simulink model "hex_simplify_mono"  (R2017a)
settings: Solver=VariableStepAuto  StartTime=0.0  StopTime=30  RelTol=1e-3
model workspace: external: MATLAB File C:\Users\laure\Documents\Gonzalo\Robotica-II\hexapod-robot\simscape\simplify_model\hex_DataFile1.m (data not in the file)
undefined symbols (not defined in the file): sigbuilder_block, smiData, X, Y, Z
libraries: sm_lib x20, nesl_utility x19
settings Model: Creator=laure  LastModifiedBy=laure

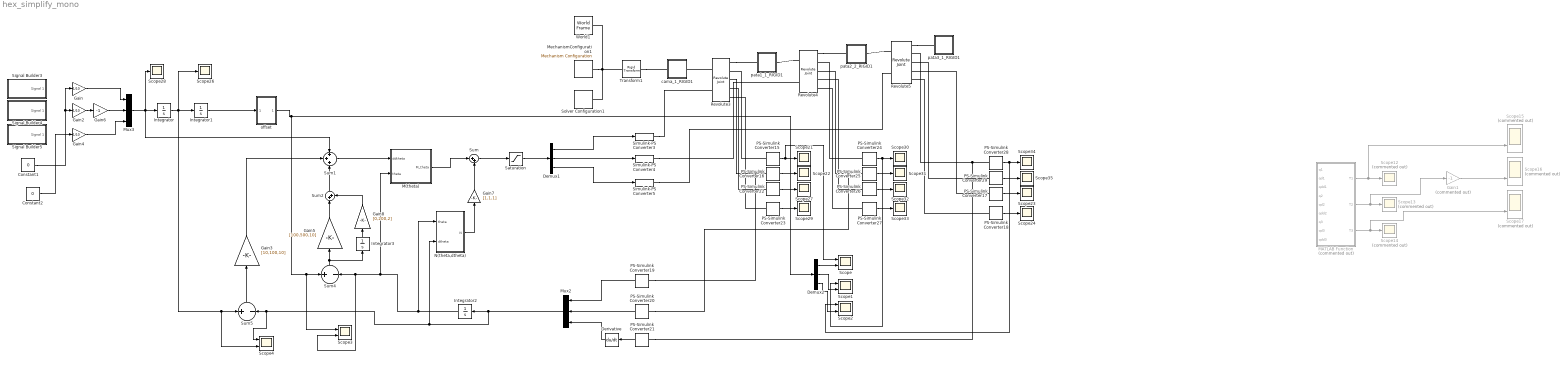
== system hex_simplify_mono ==
  Constant1 : Constant  Value=0
  Constant2 : Constant  Value=0
  Demux1 : Demux  Outputs=3
  Demux2 : Demux  Outputs=3
  Derivative : Derivative
  Gain : Gain  Gain=1/10
  Gain1 : Gain  Commented=on  Gain=-1
  Gain2 : Gain  Gain=1/10
  Gain3 : Gain  Gain=[10,100,10]
  Gain4 : Gain  Gain=1/10
  Gain5 : Gain  Gain=[100,500,10]
  Gain6 : Gain  Gain=-1
  Gain7 : Gain  Gain=[1,1,1]
  Gain8 : Gain  Gain=[0,200,2]
  Integrator : Integrator
  Integrator1 : Integrator
  Integrator2 : Integrator  InitialCondition=[-pi/2 - pi/6,-pi/2,pi/2]
  Integrator3 : Integrator  InitialCondition=[-pi/2 - pi/6,-pi/2,pi/2]
  M(theta) : Subsystem
  MATLAB Function : MATLAB Function  Commented=on  TreatAsAtomicUnit=on
  MechanismConfiguration1 : sm_lib/Utilities/Mechanism Configuration  UniformGravity=Constant  GravityVector=[0 0 -9.81]  GravityUnits=m/s^2  LinearizationDelta=0.001
  Mux2 : Mux  Inputs=3
  Mux3 : Mux  Inputs=3
  N(theta,dtheta) : Subsystem
  PS-Simulink Converter{15..29} (15 alike) : nesl_utility/PS-Simulink Converter  PhysicalDomain=network_engine_domain  SubClassName=ps_output  LeftPortType=input  RightPortType=output  PseudoPeriodic=off  Frequencies=[]  Unit=1  AffineConversion=off
  Revolute3 : sm_lib/Joints/Revolute Joint  SenseConstraintForce=off  SenseConstraintForceX=off  SenseConstraintForceY=off  SenseConstraintForceZ=off  SenseConstraintTorque=off  SenseConstraintTorqueX=off  SenseConstraintTorqueY=off  SenseConstraintTorqueZ=off  SenseTotalForce=off  SenseTotalForceX=off  SenseTotalForceY=off  SenseTotalForceZ=off  SenseTotalTorque=off  SenseTotalTorqueX=off  SenseTotalTorqueY=off  SenseTotalTorqueZ=off  CompositeWrenchDir=FollowerOnBase  CompositeWrenchFrame=BaseFrame  EquilibriumPosition=0  EquilibriumPositionUnits=rad  SpringStiffness=0  SpringStiffnessUnits=N*m/rad  DampingCoefficient=0.1  DampingCoefficientUnits=N*m/(rad/s)  TorqueActuationMode=InputTorque  MotionActuationMode=ComputedMotion  SensePosition=on  SenseVelocity=on  SenseAcceleration=on  SenseTorqueForce=on  PositionTargetSpecify=on  PositionTargetPriority=Low  PositionTargetValue=-pi/2 - pi/6  PositionTargetValueUnits=rad  VelocityTargetSpecify=off  VelocityTargetPriority=High  VelocityTargetValue=0  VelocityTargetValueUnits=deg/s
  Revolute4 : sm_lib/Joints/Revolute Joint  SenseConstraintForce=off  SenseConstraintForceX=off  SenseConstraintForceY=off  SenseConstraintForceZ=off  SenseConstraintTorque=off  SenseConstraintTorqueX=off  SenseConstraintTorqueY=off  SenseConstraintTorqueZ=off  SenseTotalForce=off  SenseTotalForceX=off  SenseTotalForceY=off  SenseTotalForceZ=off  SenseTotalTorque=off  SenseTotalTorqueX=off  SenseTotalTorqueY=off  SenseTotalTorqueZ=off  CompositeWrenchDir=FollowerOnBase  CompositeWrenchFrame=BaseFrame  EquilibriumPosition=0  EquilibriumPositionUnits=rad  SpringStiffness=0  SpringStiffnessUnits=N*m/rad  DampingCoefficient=0.1  DampingCoefficientUnits=N*m/(rad/s)  TorqueActuationMode=InputTorque  MotionActuationMode=ComputedMotion  SensePosition=on  SenseVelocity=on  SenseAcceleration=on  SenseTorqueForce=on  PositionTargetSpecify=on  PositionTargetPriority=Low  PositionTargetValue=-pi/2  PositionTargetValueUnits=rad  VelocityTargetSpecify=on  VelocityTargetPriority=High  VelocityTargetValue=0  VelocityTargetValueUnits=deg/s
  Revolute5 : sm_lib/Joints/Revolute Joint  SenseConstraintForce=off  SenseConstraintForceX=off  SenseConstraintForceY=off  SenseConstraintForceZ=off  SenseConstraintTorque=off  SenseConstraintTorqueX=off  SenseConstraintTorqueY=off  SenseConstraintTorqueZ=off  SenseTotalForce=off  SenseTotalForceX=off  SenseTotalForceY=off  SenseTotalForceZ=off  SenseTotalTorque=off  SenseTotalTorqueX=off  SenseTotalTorqueY=off  SenseTotalTorqueZ=off  CompositeWrenchDir=FollowerOnBase  CompositeWrenchFrame=BaseFrame  EquilibriumPosition=0  EquilibriumPositionUnits=rad  SpringStiffness=0  SpringStiffnessUnits=N*m/rad  DampingCoefficient=0.1  DampingCoefficientUnits=N*m/(rad/s)  TorqueActuationMode=InputTorque  MotionActuationMode=ComputedMotion  SensePosition=on  SenseVelocity=on  SenseAcceleration=on  SenseTorqueForce=on  PositionTargetSpecify=on  PositionTargetPriority=Low  PositionTargetValue=pi/2  PositionTargetValueUnits=rad  VelocityTargetSpecify=off  VelocityTargetPriority=High  VelocityTargetValue=0  VelocityTargetValueUnits=deg/s
  Saturation : Saturate  UpperLimit=5  LowerLimit=-5  LinearizeAsGain=off  ZeroCross=off
  Scope{,1..4} (5 alike) : Scope  NumInputPorts=2
  Scope12 : Scope  Commented=on
  Scope13 : Scope  Commented=on
  Scope14 : Scope  Commented=on
  Scope15 : Scope  Commented=on  NumInputPorts=2
  Scope16 : Scope  Commented=on  NumInputPorts=2
  Scope17 : Scope  Commented=on  NumInputPorts=2
  Scope{21..24,26..35} (14 alike) : Scope
  Signal Builder3 : Subsystem  Tag=STV Subsys  LoadFcn=sigbuilder_block('load');  StartFcn=sigbuilder_block('start');  StopFcn=sigbuilder_block('stop');  ClipboardFcn=sigbuilder_block('clipboard');  mask(Sigbuilder block){tuvar=[0:10]}
      mask help: Simulink:masks:SigbuilderBlock_MD
      mask init:
      | if ~strcmp(get_param(bdroot(gcbh),'SimulationStatus'),'stopped') tuvar = sigbuilder_block('maskInit'); end
      settings: CopyFcn=sigbuilder_block('copy');  DeleteFcn=sigbuilder_block('delete');  ModelCloseFcn=sigbuilder_block('modelClose');  PreSaveFcn=sigbuilder_block('preSave');  PauseFcn=sigbuilder_block('pause');  ContinueFcn=sigbuilder_block('continue');  NameChangeFcn=sigbuilder_block('namechange');  OpenFcn=sigbuilder_block('open',[319.5 111 550.5 359.25 ]);  CloseFcn=sigbuilder_block('close');
      mask Display: plot(0, 0, 100, 100,[2, 2, 32, 32, 2], [68, 8, 8, 68, 68],[32, 2], [38, 38], [32, 19, 2],[53, 60, 44], [32, 17, 17, 2],[16, 16, 31, 31]);txt = getActiveGroup(gcbh);text(2, 100, txt,'verticalAlignment', 'top');
  Signal Builder4 : Subsystem  Tag=STV Subsys  LoadFcn=sigbuilder_block('load');  StartFcn=sigbuilder_block('start');  StopFcn=sigbuilder_block('stop');  ClipboardFcn=sigbuilder_block('clipboard');  mask(Sigbuilder block){tuvar=[0:10]}
      mask help: Simulink:masks:SigbuilderBlock_MD
      mask init:
      | if ~strcmp(get_param(bdroot(gcbh),'SimulationStatus'),'stopped') tuvar = sigbuilder_block('maskInit'); end
      settings: CopyFcn=sigbuilder_block('copy');  DeleteFcn=sigbuilder_block('delete');  ModelCloseFcn=sigbuilder_block('modelClose');  PreSaveFcn=sigbuilder_block('preSave');  PauseFcn=sigbuilder_block('pause');  ContinueFcn=sigbuilder_block('continue');  NameChangeFcn=sigbuilder_block('namechange');  OpenFcn=sigbuilder_block('open',[319.5 111 550.5 359.25 ]);  CloseFcn=sigbuilder_block('close');
      mask Display: plot(0, 0, 100, 100,[2, 2, 32, 32, 2], [68, 8, 8, 68, 68],[32, 2], [38, 38], [32, 19, 2],[53, 60, 44], [32, 17, 17, 2],[16, 16, 31, 31]);txt = getActiveGroup(gcbh);text(2, 100, txt,'verticalAlignment', 'top');
  Signal Builder5 : Subsystem  Tag=STV Subsys  LoadFcn=sigbuilder_block('load');  StartFcn=sigbuilder_block('start');  StopFcn=sigbuilder_block('stop');  ClipboardFcn=sigbuilder_block('clipboard');  mask(Sigbuilder block){tuvar=[0:10]}
      mask help: Simulink:masks:SigbuilderBlock_MD
      mask init:
      | if ~strcmp(get_param(bdroot(gcbh),'SimulationStatus'),'stopped') tuvar = sigbuilder_block('maskInit'); end
      settings: CopyFcn=sigbuilder_block('copy');  DeleteFcn=sigbuilder_block('delete');  ModelCloseFcn=sigbuilder_block('modelClose');  PreSaveFcn=sigbuilder_block('preSave');  PauseFcn=sigbuilder_block('pause');  ContinueFcn=sigbuilder_block('continue');  NameChangeFcn=sigbuilder_block('namechange');  OpenFcn=sigbuilder_block('open',[319.5 111 550.5 359.25 ]);  CloseFcn=sigbuilder_block('close');
      mask Display: plot(0, 0, 100, 100,[2, 2, 32, 32, 2], [68, 8, 8, 68, 68],[32, 2], [38, 38], [32, 19, 2],[53, 60, 44], [32, 17, 17, 2],[16, 16, 31, 31]);txt = getActiveGroup(gcbh);text(2, 100, txt,'verticalAlignment', 'top');
  Simulink-PS Converter3 : nesl_utility/Simulink-PS Converter  PhysicalDomain=network_engine_domain  SubClassName=ps_input  LeftPortType=input  RightPortType=output  PseudoPeriodic=off  Frequencies=[]  NoiseDistribution=none  NoiseParameters=[]  Unit=1  AffineConversion=off  FilteringAndDerivatives=filter  SimscapeFilterOrder=2  InputFilterTimeConstant=0.001  UdotUserProvided=0
  Simulink-PS Converter4 : nesl_utility/Simulink-PS Converter  PhysicalDomain=network_engine_domain  SubClassName=ps_input  LeftPortType=input  RightPortType=output  PseudoPeriodic=off  Frequencies=[]  NoiseDistribution=none  NoiseParameters=[]  Unit=1  AffineConversion=off  FilteringAndDerivatives=filter  SimscapeFilterOrder=2  InputFilterTimeConstant=0.001  UdotUserProvided=0
  Simulink-PS Converter5 : nesl_utility/Simulink-PS Converter  PhysicalDomain=network_engine_domain  SubClassName=ps_input  LeftPortType=input  RightPortType=output  PseudoPeriodic=off  Frequencies=[]  NoiseDistribution=none  NoiseParameters=[]  Unit=1  AffineConversion=off  FilteringAndDerivatives=filter  SimscapeFilterOrder=2  InputFilterTimeConstant=0.001  UdotUserProvided=0
  Solver Configuration1 : nesl_utility/Solver Configuration  PhysicalDomain=network_engine_domain  SubClassName=solver  LeftPortType=input  RightPortType=generic  Accelerate=off  Tones=[]  Harmonics=[]  SimulateNoise=off  Profile=off  UseLocalSampling=off  EnableSwitchedLinearOptims=on  FrequencyDomain=off  UseCCode=off  RelTol=0.001  AbsTol=1e-06  MinStep=1e-09  ToWorkspace=off  RevertToSquareIcSolve=off  NumHomotopyIterations=100  PhasorMode=off  PhasorModeNumHarmonics=1  OverrideAbsTol=off  DoDC=off  ResidualTolerance=1e-09  UseLocalSolver=off  LocalSolverChoice=NE_BACKWARD_EULER_ADVANCER  LocalSolverSampleTime=0.001  DoFixedCost=off  MaxNonlinIter=3  MaxModeIter=2  LinearAlgebra=Sparse  DelaysMemoryBudget=1024  AutomaticFiltering=on  FilteringTimeConstant=0.001
  Sum : Sum  Inputs=|++
  Sum1 : Sum  Inputs=+++
  Sum2 : Sum  Inputs=|++
  Sum4 : Sum  Inputs=+-
  Sum5 : Sum  Inputs=+-
  Transform1 : sm_lib/Frames and Transforms/Rigid Transform  TranslationMethod=Cartesian  TranslationStandardOffset=0  TranslationLengthUnit=mm  TranslationStandardAxis=+Z  TranslationCartesianOffset=smiData.RigidTransform(7).translation  TranslationROffset=0  TranslationROffsetUnits=m  TranslationZOffset=0  TranslationZOffsetUnits=m  TranslationThetaOffset=0  TranslationThetaOffsetUnits=deg  RotationMethod=ArbitraryAxis  RotationAngleUnits=rad  RotationStandardAxis=+Z  RotationAngle=smiData.RigidTransform(7).angle  RotationArbitraryAxis=smiData.RigidTransform(7).axis  FollAlignAxisA=+X  BaseAlignAxisA=+Y  FollAlignAxisB=+Y  BaseAlignAxisB=+Z  RotationSequenceAxes=FollowerAxes  RotationSequence=XYX  RotationSequenceAngles=[0 0 0]  RotationSequenceAnglesUnits=deg  RotationMatrix=[1 0 0; 0 1 0; 0 0 1]
  World1 : sm_lib/Frames and Transforms/World Frame
  cama_1_RIGID1 : Subsystem
  "offset " : Subsystem
  pata1_1_RIGID1 : Subsystem
  pata2_2_RIGID1 : Subsystem
  pata3_1_RIGID1 : Subsystem
  wires:
  MATLAB Function/1(T1) -> Scope15/2, Scope12/1
  MATLAB Function/3(T3) -> Scope17/2, Scope14/1
  MATLAB Function/2(T2) -> Gain1/1, Scope13/1
  Gain1/1 -> Scope16/2
  Gain6/1 -> Mux3/2
  Sum5/1 -> Gain3/1
  Gain/1 -> Mux3/1
  Integrator1/1 -> "offset "/1(In1)
  PS-Simulink Converter19/1 -> Mux2/1
  PS-Simulink Converter21/1 -> Derivative/1
  Mux3/1 -> Sum1/1, Integrator/1, Scope28/1
  PS-Simulink Converter18/1 -> Scope24/1
  PS-Simulink Converter28/1 -> Scope2/1, Scope34/1
  Sum4/1 -> Gain5/1, Integrator3/1
  PS-Simulink Converter29/1 -> Scope35/1
  PS-Simulink Converter25/1 -> Scope31/1
  PS-Simulink Converter20/1 -> Mux2/2
  PS-Simulink Converter24/1 -> Scope1/1, Scope30/1
  PS-Simulink Converter26/1 -> Scope32/1
  Integrator/1 -> Integrator1/1, Scope4/2, Sum5/1, Scope26/1
  PS-Simulink Converter27/1 -> Scope33/1
  PS-Simulink Converter16/1 -> Scope22/1
  PS-Simulink Converter23/1 -> Scope29/1
  PS-Simulink Converter22/1 -> Scope27/1
  Gain4/1 -> Mux3/3
  PS-Simulink Converter15/1 -> Scope/1, Scope21/1
  PS-Simulink Converter17/1 -> Scope23/1
  Gain2/1 -> Gain6/1
  "offset "/1(Out1) -> Scope3/1, Sum4/1, Demux2/1
  Sum/1 -> Saturation/1
  N(theta,dtheta)/1(N) -> Gain7/1
  Gain3/1 -> Sum1/2
  Demux2/1 -> Scope/2
  Demux2/2 -> Scope1/2
  Demux2/3 -> Scope2/2
  Sum1/1 -> M(theta)/1(ddtheta)
  M(theta)/1(M_theta) -> Sum/1
  Gain7/1 -> Sum/2
  Mux2/1 -> N(theta,dtheta)/2(dtheta), Scope4/1, Sum5/2, Integrator2/1
  Integrator2/1 -> N(theta,dtheta)/1(theta), M(theta)/2(theta), Scope3/2, Sum4/2
  Demux1/1 -> Simulink-PS Converter3/1
  Demux1/2 -> Simulink-PS Converter4/1
  Sum2/1 -> Sum1/3
  Gain5/1 -> Sum2/1
  Integrator3/1 -> Gain8/1
  Gain8/1 -> Sum2/2
  Derivative/1 -> Mux2/3
  Saturation/1 -> Demux1/1
  Demux1/3 -> Simulink-PS Converter5/1
  Constant1/1 -> Gain2/1, Gain/1
  Constant2/1 -> Gain4/1
  connections:
  World1/RConn1 -- Transform1/LConn1 -- MechanismConfiguration1/RConn1 -- Solver Configuration1/RConn1
  PS-Simulink Converter28/LConn1 -- PS-Simulink Converter21/LConn1 -- Revolute5/RConn2
  PS-Simulink Converter15/LConn1 -- Revolute3/RConn2
  PS-Simulink Converter24/LConn1 -- Revolute4/RConn2
  Revolute4/RConn1 -- pata2_2_RIGID1/LConn1
  PS-Simulink Converter22/LConn1 -- Revolute3/RConn4
  PS-Simulink Converter17/LConn1 -- Revolute5/RConn4
  Transform1/RConn1 -- cama_1_RIGID1/LConn1
  PS-Simulink Converter23/LConn1 -- Revolute3/RConn5
  Simulink-PS Converter5/RConn1 -- Revolute5/LConn2
  PS-Simulink Converter25/LConn1 -- PS-Simulink Converter20/LConn1 -- Revolute4/RConn3
  PS-Simulink Converter27/LConn1 -- Revolute4/RConn5
  PS-Simulink Converter26/LConn1 -- Revolute4/RConn4
  Revolute3/LConn1 -- cama_1_RIGID1/RConn1
  Revolute4/LConn1 -- pata1_1_RIGID1/RConn1
  Revolute5/RConn1 -- pata3_1_RIGID1/LConn1
  Revolute5/LConn1 -- pata2_2_RIGID1/RConn1
  Simulink-PS Converter3/RConn1 -- Revolute3/LConn2
  PS-Simulink Converter18/LConn1 -- Revolute5/RConn5
  PS-Simulink Converter29/LConn1 -- Revolute5/RConn3
  Simulink-PS Converter4/RConn1 -- Revolute4/LConn2
  Revolute3/RConn1 -- pata1_1_RIGID1/LConn1
  Revolute3/RConn3 -- PS-Simulink Converter19/LConn1 -- PS-Simulink Converter16/LConn1

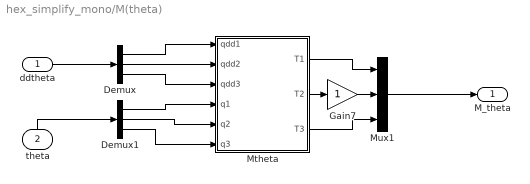
== system hex_simplify_mono/M(theta) ==
  ddtheta : Inport
  theta : Inport  Port=2
  Demux : Demux  Outputs=3
  Demux1 : Demux  Outputs=3
  Gain7 : Gain
  Mtheta : MATLAB Function  TreatAsAtomicUnit=on
  Mux1 : Mux  Inputs=3
  M_theta : Outport
  wires:
  Mux1/1 -> M_theta/1
  Mtheta/3(T3) -> Mux1/3
  Mtheta/2(T2) -> Gain7/1
  Mtheta/1(T1) -> Mux1/1
  Gain7/1 -> Mux1/2
  ddtheta/1 -> Demux/1
  theta/1 -> Demux1/1
  Demux/2 -> Mtheta/2(qdd2)
  Demux/1 -> Mtheta/1(qdd1)
  Demux/3 -> Mtheta/3(qdd3)
  Demux1/1 -> Mtheta/4(q1)
  Demux1/2 -> Mtheta/5(q2)
  Demux1/3 -> Mtheta/6(q3)

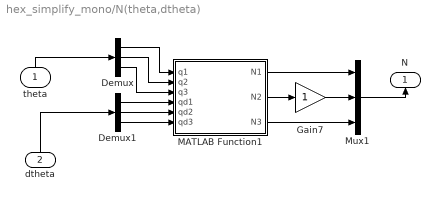
== system hex_simplify_mono/N(theta,dtheta) ==
  theta : Inport
  dtheta : Inport  Port=2
  Demux : Demux  Outputs=3
  Demux1 : Demux  Outputs=3
  Gain7 : Gain
  MATLAB Function1 : MATLAB Function  TreatAsAtomicUnit=on
  Mux1 : Mux  Inputs=3
  N : Outport
  wires:
  MATLAB Function1/3(N3) -> Mux1/3
  MATLAB Function1/1(N1) -> Mux1/1
  Mux1/1 -> N/1
  MATLAB Function1/2(N2) -> Gain7/1
  theta/1 -> Demux/1
  dtheta/1 -> Demux1/1
  Demux/1 -> MATLAB Function1/1(q1)
  Demux/2 -> MATLAB Function1/2(q2)
  Demux/3 -> MATLAB Function1/3(q3)
  Demux1/1 -> MATLAB Function1/4(qd1)
  Demux1/2 -> MATLAB Function1/5(qd2)
  Demux1/3 -> MATLAB Function1/6(qd3)
  Gain7/1 -> Mux1/2

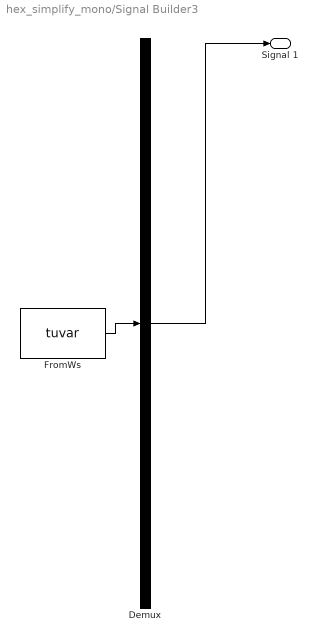
== system hex_simplify_mono/Signal Builder3 ==
  Demux : Demux  Tag=STV Demux  Outputs=1
  FromWs : FromWorkspace  Tag=STV FromWs  VariableName=tuvar  SampleTime=0
      SigBuilderData=|
      | common.afterFinalStr = 'Extrapolate'
      | common.sampleTime = 0
      | dataSet.timeRange = [0 10]
      | dataSet.name = 'Group 1'
      | sbobj.Groups.Name = 'Group 1'
      | sbobj.Groups.Signals.Name = 'Signal 1'
      | sbobj.Groups.Signals.XData = [0 4 6 10]
      | sbobj.Groups.Signals.YData = [0 1.57079632679 1.57079632679 0]
  Signal 1 : Outport  Tag=STV Outport
  wires:
  Demux/1 -> Signal 1/1
  FromWs/1 -> Demux/1

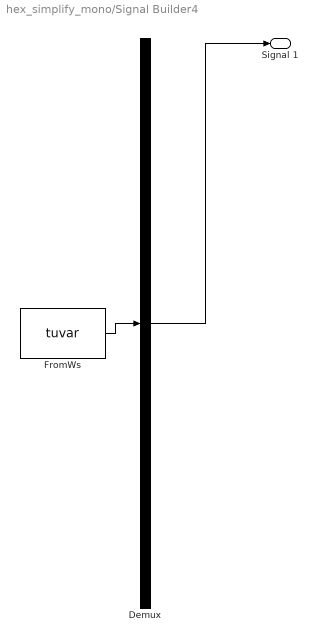
== system hex_simplify_mono/Signal Builder4 ==
  Demux : Demux  Tag=STV Demux  Outputs=1
  FromWs : FromWorkspace  Tag=STV FromWs  VariableName=tuvar  SampleTime=0
      SigBuilderData=|
      | common.afterFinalStr = 'Extrapolate'
      | common.sampleTime = 0
      | dataSet.timeRange = [0 10]
      | dataSet.name = 'Group 1'
      | sbobj.Groups.Name = 'Group 1'
      | sbobj.Groups.Signals.Name = 'Signal 1'
      | sbobj.Groups.Signals.XData = [0 4 6 10]
      | sbobj.Groups.Signals.YData = [0 1.57079632679 1.57079632679 0]
  Signal 1 : Outport  Tag=STV Outport
  wires:
  Demux/1 -> Signal 1/1
  FromWs/1 -> Demux/1

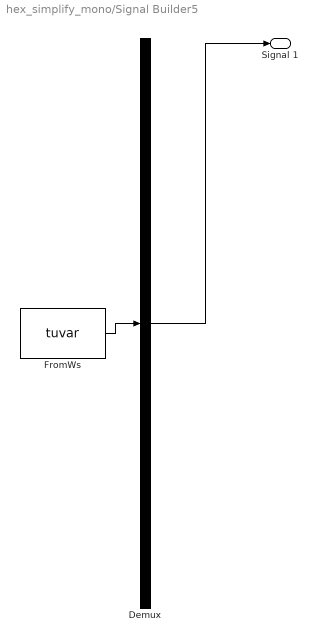
== system hex_simplify_mono/Signal Builder5 ==
  Demux : Demux  Tag=STV Demux  Outputs=1
  FromWs : FromWorkspace  Tag=STV FromWs  VariableName=tuvar  SampleTime=0
      SigBuilderData=|
      | common.afterFinalStr = 'Extrapolate'
      | common.sampleTime = 0
      | dataSet.timeRange = [0 10]
      | dataSet.name = 'Group 1'
      | sbobj.Groups.Name = 'Group 1'
      | sbobj.Groups.Signals.Name = 'Signal 1'
      | sbobj.Groups.Signals.XData = [0 4 6 10]
      | sbobj.Groups.Signals.YData = [0 1.57079632679 1.57079632679 0]
  Signal 1 : Outport  Tag=STV Outport
  wires:
  Demux/1 -> Signal 1/1
  FromWs/1 -> Demux/1

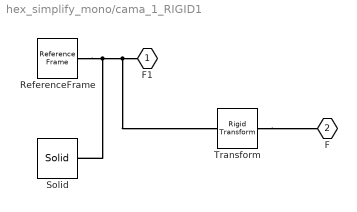
== system hex_simplify_mono/cama_1_RIGID1 ==
  ReferenceFrame : sm_lib/Frames and Transforms/Reference Frame
  Solid : sm_lib/Body Elements/Solid  InertiaType=Custom  Mass=smiData.Solid(2).mass  MassUnits=kg  CenterOfMass=smiData.Solid(2).CoM  CenterOfMassUnits=mm  MomentsOfInertia=smiData.Solid(2).MoI  MomentsOfInertiaUnits=kg*mm^2  ProductsOfInertia=smiData.Solid(2).PoI  ProductsOfInertiaUnits=kg*mm^2  DensityBased=on  Density=1000  DensityUnits=kg/m^3  DoExposeReferenceFrame=on  SerializedFrames=<Frames/>  GraphicType=FromGeometry  MarkerShape=Sphere  MarkerSize=10  GraphicVisPropType=SimpleVisualProperties  GraphicDiffuseColor=smiData.Solid(2).color  GraphicSpecularColor=[0.5 0.5 0.5 1.0]  GraphicAmbientColor=[0.15 0.15 0.15 1.0]  GraphicEmissiveColor=[0.0 0.0 0.0 1.0]  GraphicShininess=75  GraphicOpacity=smiData.Solid(2).opacity  GeometryShape=FromFile  RectangleSize=[1 1]  RectangleSizeUnits=m  BrickDimensions=[1 1 1]  BrickDimensionUnits=m  CylinderRadius=1  CylinderRadiusUnits=m  CylinderLength=1  CylinderLengthUnits=m  SphereRadius=1  SphereRadiusUnits=m  EllipsoidRadii=[1 1 1]  EllipsoidRadiiUnits=m  ExtrusionCrossSection=[1 1; -1 1; -1 -1; 1 -1]  ExtrusionCrossSectionUnits=m  ExtrusionLength=1  ExtrusionLengthUnits=m  PolygonNumSides=3  PolygonOuterRadius=1  PolygonOuterRadiusUnits=m  ExtGeomFileType=STEP  ExtGeomFileName=cama_Predeterminado_sldprt.STEP  ExtGeomFileUnits=m  RevolutionCrossSection=[1 1; 1 -1; 2 -1; 2 1]  RevolutionCrossSectionUnits=m  RevolutionExtent=Full  RevolutionAngle=180  RevolutionAngleUnits=deg
  Transform : sm_lib/Frames and Transforms/Rigid Transform  TranslationMethod=Cartesian  TranslationStandardOffset=0  TranslationLengthUnit=mm  TranslationStandardAxis=+Z  TranslationCartesianOffset=smiData.RigidTransform(1).translation  TranslationROffset=0  TranslationROffsetUnits=m  TranslationZOffset=0  TranslationZOffsetUnits=m  TranslationThetaOffset=0  TranslationThetaOffsetUnits=deg  RotationMethod=ArbitraryAxis  RotationAngleUnits=rad  RotationStandardAxis=+Z  RotationAngle=smiData.RigidTransform(1).angle  RotationArbitraryAxis=smiData.RigidTransform(1).axis  FollAlignAxisA=+X  BaseAlignAxisA=+Y  FollAlignAxisB=+Y  BaseAlignAxisB=+Z  RotationSequenceAxes=FollowerAxes  RotationSequence=XYX  RotationSequenceAngles=[0 0 0]  RotationSequenceAnglesUnits=deg  RotationMatrix=[1 0 0; 0 1 0; 0 0 1]
  F1 : PMIOPort  Port=1  Side=Left
  F : PMIOPort  Port=2  Side=Right
  connections:
  Solid/RConn1 -- ReferenceFrame/RConn1 -- Transform/LConn1 -- F1/RConn1
  Transform/RConn1 -- F/RConn1

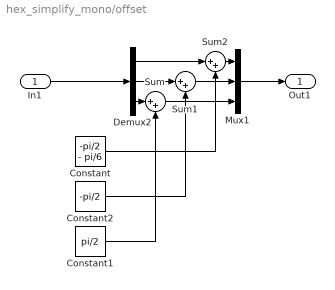
== system hex_simplify_mono/offset  ==
  In1 : Inport
  Constant : Constant  Value=-pi/2 - pi/6
  Constant1 : Constant  Value=pi/2
  Constant2 : Constant  Value=-pi/2
  Demux2 : Demux  Outputs=3
  Mux1 : Mux  Inputs=3
  Sum : Sum  Inputs=|++
  Sum1 : Sum  Inputs=|++
  Sum2 : Sum  Inputs=|++
  Out1 : Outport
  wires:
  Mux1/1 -> Out1/1
  In1/1 -> Demux2/1
  Sum/1 -> Mux1/3
  Demux2/3 -> Sum/1
  Sum1/1 -> Mux1/2
  Demux2/2 -> Sum1/1
  Sum2/1 -> Mux1/1
  Demux2/1 -> Sum2/1
  Constant/1 -> Sum2/2
  Constant2/1 -> Sum1/2
  Constant1/1 -> Sum/2

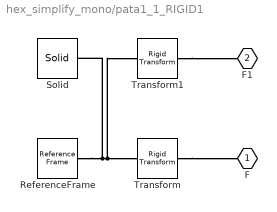
== system hex_simplify_mono/pata1_1_RIGID1 ==
  ReferenceFrame : sm_lib/Frames and Transforms/Reference Frame
  Solid : sm_lib/Body Elements/Solid  InertiaType=Custom  Mass=2  MassUnits=kg  CenterOfMass=[24.25,7.5,-7.5]  CenterOfMassUnits=mm  MomentsOfInertia=[0,0,0]  MomentsOfInertiaUnits=kg*mm^2  ProductsOfInertia=[0,0,0]  ProductsOfInertiaUnits=kg*mm^2  DensityBased=on  Density=1000  DensityUnits=kg/m^3  DoExposeReferenceFrame=on  SerializedFrames=<Frames/>  GraphicType=FromGeometry  MarkerShape=Sphere  MarkerSize=10  GraphicVisPropType=SimpleVisualProperties  GraphicDiffuseColor=smiData.Solid(4).color  GraphicSpecularColor=[0.5 0.5 0.5 1.0]  GraphicAmbientColor=[0.15 0.15 0.15 1.0]  GraphicEmissiveColor=[0.0 0.0 0.0 1.0]  GraphicShininess=75  GraphicOpacity=smiData.Solid(4).opacity  GeometryShape=FromFile  RectangleSize=[1 1]  RectangleSizeUnits=m  BrickDimensions=[1 1 1]  BrickDimensionUnits=m  CylinderRadius=1  CylinderRadiusUnits=m  CylinderLength=1  CylinderLengthUnits=m  SphereRadius=1  SphereRadiusUnits=m  EllipsoidRadii=[1 1 1]  EllipsoidRadiiUnits=m  ExtrusionCrossSection=[1 1; -1 1; -1 -1; 1 -1]  ExtrusionCrossSectionUnits=m  ExtrusionLength=1  ExtrusionLengthUnits=m  PolygonNumSides=3  PolygonOuterRadius=1  PolygonOuterRadiusUnits=m  ExtGeomFileType=STEP  ExtGeomFileName=pata1_Predeterminado_sldprt.STEP  ExtGeomFileUnits=m  RevolutionCrossSection=[1 1; 1 -1; 2 -1; 2 1]  RevolutionCrossSectionUnits=m  RevolutionExtent=Full  RevolutionAngle=180  RevolutionAngleUnits=deg
  Transform : sm_lib/Frames and Transforms/Rigid Transform  TranslationMethod=Cartesian  TranslationStandardOffset=0  TranslationLengthUnit=mm  TranslationStandardAxis=+Z  TranslationCartesianOffset=smiData.RigidTransform(2).translation  TranslationROffset=0  TranslationROffsetUnits=m  TranslationZOffset=0  TranslationZOffsetUnits=m  TranslationThetaOffset=0  TranslationThetaOffsetUnits=deg  RotationMethod=ArbitraryAxis  RotationAngleUnits=rad  RotationStandardAxis=+Z  RotationAngle=smiData.RigidTransform(2).angle  RotationArbitraryAxis=smiData.RigidTransform(2).axis  FollAlignAxisA=+X  BaseAlignAxisA=+Y  FollAlignAxisB=+Y  BaseAlignAxisB=+Z  RotationSequenceAxes=FollowerAxes  RotationSequence=XYX  RotationSequenceAngles=[0 0 0]  RotationSequenceAnglesUnits=deg  RotationMatrix=[1 0 0; 0 1 0; 0 0 1]
  Transform1 : sm_lib/Frames and Transforms/Rigid Transform  TranslationMethod=Cartesian  TranslationStandardOffset=0  TranslationLengthUnit=mm  TranslationStandardAxis=+Z  TranslationCartesianOffset=smiData.RigidTransform(3).translation  TranslationROffset=0  TranslationROffsetUnits=m  TranslationZOffset=0  TranslationZOffsetUnits=m  TranslationThetaOffset=0  TranslationThetaOffsetUnits=deg  RotationMethod=ArbitraryAxis  RotationAngleUnits=rad  RotationStandardAxis=+Z  RotationAngle=smiData.RigidTransform(3).angle  RotationArbitraryAxis=smiData.RigidTransform(3).axis  FollAlignAxisA=+X  BaseAlignAxisA=+Y  FollAlignAxisB=+Y  BaseAlignAxisB=+Z  RotationSequenceAxes=FollowerAxes  RotationSequence=XYX  RotationSequenceAngles=[0 0 0]  RotationSequenceAnglesUnits=deg  RotationMatrix=[1 0 0; 0 1 0; 0 0 1]
  F : PMIOPort  Port=1  Side=Left
  F1 : PMIOPort  Port=2  Side=Right
  connections:
  Solid/RConn1 -- ReferenceFrame/RConn1 -- Transform/LConn1 -- Transform1/LConn1
  Transform/RConn1 -- F/RConn1
  Transform1/RConn1 -- F1/RConn1

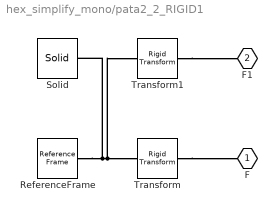
== system hex_simplify_mono/pata2_2_RIGID1 ==
  ReferenceFrame : sm_lib/Frames and Transforms/Reference Frame
  Solid : sm_lib/Body Elements/Solid  InertiaType=Custom  Mass=2  MassUnits=kg  CenterOfMass=[47.9, 7.5, 12.5]  CenterOfMassUnits=mm  MomentsOfInertia=[0,0,0]  MomentsOfInertiaUnits=kg*mm^2  ProductsOfInertia=[0,0,0]  ProductsOfInertiaUnits=kg*mm^2  DensityBased=on  Density=1000  DensityUnits=kg/m^3  DoExposeReferenceFrame=on  SerializedFrames=<Frames/>  GraphicType=FromGeometry  MarkerShape=Sphere  MarkerSize=10  GraphicVisPropType=SimpleVisualProperties  GraphicDiffuseColor=smiData.Solid(3).color  GraphicSpecularColor=[0.5 0.5 0.5 1.0]  GraphicAmbientColor=[0.15 0.15 0.15 1.0]  GraphicEmissiveColor=[0.0 0.0 0.0 1.0]  GraphicShininess=75  GraphicOpacity=smiData.Solid(3).opacity  GeometryShape=FromFile  RectangleSize=[1 1]  RectangleSizeUnits=m  BrickDimensions=[1 1 1]  BrickDimensionUnits=m  CylinderRadius=1  CylinderRadiusUnits=m  CylinderLength=1  CylinderLengthUnits=m  SphereRadius=1  SphereRadiusUnits=m  EllipsoidRadii=[1 1 1]  EllipsoidRadiiUnits=m  ExtrusionCrossSection=[1 1; -1 1; -1 -1; 1 -1]  ExtrusionCrossSectionUnits=m  ExtrusionLength=1  ExtrusionLengthUnits=m  PolygonNumSides=3  PolygonOuterRadius=1  PolygonOuterRadiusUnits=m  ExtGeomFileType=STEP  ExtGeomFileName=pata2_Predeterminado_sldprt.STEP  ExtGeomFileUnits=m  RevolutionCrossSection=[1 1; 1 -1; 2 -1; 2 1]  RevolutionCrossSectionUnits=m  RevolutionExtent=Full  RevolutionAngle=180  RevolutionAngleUnits=deg
  Transform : sm_lib/Frames and Transforms/Rigid Transform  TranslationMethod=Cartesian  TranslationStandardOffset=0  TranslationLengthUnit=mm  TranslationStandardAxis=+Z  TranslationCartesianOffset=smiData.RigidTransform(4).translation  TranslationROffset=0  TranslationROffsetUnits=m  TranslationZOffset=0  TranslationZOffsetUnits=m  TranslationThetaOffset=0  TranslationThetaOffsetUnits=deg  RotationMethod=ArbitraryAxis  RotationAngleUnits=rad  RotationStandardAxis=+Z  RotationAngle=smiData.RigidTransform(4).angle  RotationArbitraryAxis=smiData.RigidTransform(4).axis  FollAlignAxisA=+X  BaseAlignAxisA=+Y  FollAlignAxisB=+Y  BaseAlignAxisB=+Z  RotationSequenceAxes=FollowerAxes  RotationSequence=XYX  RotationSequenceAngles=[0 0 0]  RotationSequenceAnglesUnits=deg  RotationMatrix=[1 0 0; 0 1 0; 0 0 1]
  Transform1 : sm_lib/Frames and Transforms/Rigid Transform  TranslationMethod=Cartesian  TranslationStandardOffset=0  TranslationLengthUnit=mm  TranslationStandardAxis=+Z  TranslationCartesianOffset=smiData.RigidTransform(5).translation  TranslationROffset=0  TranslationROffsetUnits=m  TranslationZOffset=0  TranslationZOffsetUnits=m  TranslationThetaOffset=0  TranslationThetaOffsetUnits=deg  RotationMethod=ArbitraryAxis  RotationAngleUnits=rad  RotationStandardAxis=+Z  RotationAngle=smiData.RigidTransform(5).angle  RotationArbitraryAxis=smiData.RigidTransform(5).axis  FollAlignAxisA=+X  BaseAlignAxisA=+Y  FollAlignAxisB=+Y  BaseAlignAxisB=+Z  RotationSequenceAxes=FollowerAxes  RotationSequence=XYX  RotationSequenceAngles=[0 0 0]  RotationSequenceAnglesUnits=deg  RotationMatrix=[1 0 0; 0 1 0; 0 0 1]
  F : PMIOPort  Port=1  Side=Left
  F1 : PMIOPort  Port=2  Side=Right
  connections:
  Solid/RConn1 -- ReferenceFrame/RConn1 -- Transform/LConn1 -- Transform1/LConn1
  Transform/RConn1 -- F/RConn1
  Transform1/RConn1 -- F1/RConn1

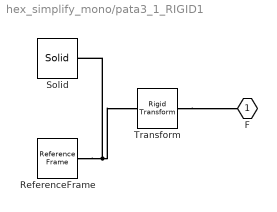
== system hex_simplify_mono/pata3_1_RIGID1 ==
  ReferenceFrame : sm_lib/Frames and Transforms/Reference Frame
  Solid : sm_lib/Body Elements/Solid  InertiaType=Custom  Mass=2  MassUnits=kg  CenterOfMass=[7.5,7.5,-10-129.8/2]  CenterOfMassUnits=mm  MomentsOfInertia=[0,0,0]  MomentsOfInertiaUnits=kg*mm^2  ProductsOfInertia=[0,0,0]  ProductsOfInertiaUnits=kg*mm^2  DensityBased=on  Density=1000  DensityUnits=kg/m^3  DoExposeReferenceFrame=on  SerializedFrames=<Frames/>  GraphicType=FromGeometry  MarkerShape=Sphere  MarkerSize=10  GraphicVisPropType=SimpleVisualProperties  GraphicDiffuseColor=smiData.Solid(1).color  GraphicSpecularColor=[0.5 0.5 0.5 1.0]  GraphicAmbientColor=[0.15 0.15 0.15 1.0]  GraphicEmissiveColor=[0.0 0.0 0.0 1.0]  GraphicShininess=75  GraphicOpacity=smiData.Solid(1).opacity  GeometryShape=FromFile  RectangleSize=[1 1]  RectangleSizeUnits=m  BrickDimensions=[1 1 1]  BrickDimensionUnits=m  CylinderRadius=1  CylinderRadiusUnits=m  CylinderLength=1  CylinderLengthUnits=m  SphereRadius=1  SphereRadiusUnits=m  EllipsoidRadii=[1 1 1]  EllipsoidRadiiUnits=m  ExtrusionCrossSection=[1 1; -1 1; -1 -1; 1 -1]  ExtrusionCrossSectionUnits=m  ExtrusionLength=1  ExtrusionLengthUnits=m  PolygonNumSides=3  PolygonOuterRadius=1  PolygonOuterRadiusUnits=m  ExtGeomFileType=STEP  ExtGeomFileName=pata3_Predeterminado_sldprt.STEP  ExtGeomFileUnits=m  RevolutionCrossSection=[1 1; 1 -1; 2 -1; 2 1]  RevolutionCrossSectionUnits=m  RevolutionExtent=Full  RevolutionAngle=180  RevolutionAngleUnits=deg
  Transform : sm_lib/Frames and Transforms/Rigid Transform  TranslationMethod=Cartesian  TranslationStandardOffset=0  TranslationLengthUnit=mm  TranslationStandardAxis=+Z  TranslationCartesianOffset=smiData.RigidTransform(6).translation  TranslationROffset=0  TranslationROffsetUnits=m  TranslationZOffset=0  TranslationZOffsetUnits=m  TranslationThetaOffset=0  TranslationThetaOffsetUnits=deg  RotationMethod=ArbitraryAxis  RotationAngleUnits=rad  RotationStandardAxis=+Z  RotationAngle=smiData.RigidTransform(6).angle  RotationArbitraryAxis=smiData.RigidTransform(6).axis  FollAlignAxisA=+X  BaseAlignAxisA=+Y  FollAlignAxisB=+Y  BaseAlignAxisB=+Z  RotationSequenceAxes=FollowerAxes  RotationSequence=XYX  RotationSequenceAngles=[0 0 0]  RotationSequenceAnglesUnits=deg  RotationMatrix=[1 0 0; 0 1 0; 0 0 1]
  F : PMIOPort  Port=1  Side=Left
  connections:
  Solid/RConn1 -- ReferenceFrame/RConn1 -- Transform/LConn1
  Transform/RConn1 -- F/RConn1

== matlab function hex_simplify_mono/M(theta)/Mtheta ==
  data: qdd1 input; T1 output; qdd2 input; T2 output; T3 output; qdd3 input; q1 input; q2 input; q3 input
function [T1, T2, T3] = fcn(qdd1,qdd2,qdd3,q1,q2,q3)

l1 = 0.0285; l2 = 0.0758; l3 = 0.1298;
lc1 = l1/2; lc2 = l2/2; lc3 = l3/2;

Ixx1 = 0.000; Ixx2 = 0.000; Ixx3 = 0.000;
Iyy1 = 0.000; Iyy2 = 0.000; Iyy3 = 0.000;
Izz1 = 0.000; Izz2 = 0.000; Izz3 = 0.0000;

gx = 0;
gy = 0;
gz = 9.81;
m1 = 2; m2 = 2; m3 = 2;

Fx = 0;
Fy = 0;
Fz = 0;
b1 = 0.1; b2 = 0.1; b3 = 0.1; 



M = [ Ixx2/2 + Ixx3/2 + Iyy1 + Iyy2/2 + Iyy3/2 - (Ixx3*cos(2*q2 + 2*q3))/2 + (Iyy3*cos(2*q2 + 2*q3))/2 + l1^2*m2 + l1^2*m3 + (l2^2*m3)/2 + lc1^2*m1 + (lc2^2*m2)/2 + (lc3^2*m3)/2 - (Ixx2*cos(2*q2))/2 + (Iyy2*cos(2*q2))/2 + (l2^2*m3*cos(2*q2))/2 + (lc2^2*m2*cos(2*q2))/2 + (lc3^2*m3*cos(2*q2 + 2*q3))/2 + 2*l1*lc3*m3*cos(q2 + q3) + 2*l1*l2*m3*cos(q2) + 2*l1*lc2*m2*cos(q2) + l2*lc3*m3*cos(q3) + l2*lc3*m3*cos(2*q2 + q3),                                                                 0,                                0;
                                                                                                                                                                                                                                                                                                                                                                                                                           0, m3*l2^2 + 2*m3*cos(q3)*l2*lc3 + m2*lc2^2 + m3*lc3^2 + Izz2 + Izz3, Izz3 + lc3*m3*(lc3 + l2*cos(q3));

                                                                                                                                                                                                                                                                                                                                                                                                                           0,                               m3*lc3^2 + l2*m3*cos(q3)*lc3 + Izz3,                  m3*lc3^2 + Izz3];

                                                                                                                                                                                                                                                                                                                                                                                                                       
 T1 = M(1, 1) * qdd1 + M(1, 2) * qdd2 + M(1, 3) * qdd3;
 T2 = M(2, 1) * qdd1 + M(2, 2) * qdd2 + M(2, 3) * qdd3;
 T3 = M(3, 1) * qdd1 + M(3, 2) * qdd2 + M(3, 3) * qdd3;

== matlab function hex_simplify_mono/MATLAB Function ==
  data: T1 output; T2 output; T3 output; q1 input; qd1 input; qdd1 input; q2 input; qd2 input; qdd2 input; q3 input; qd3 input; qdd3 input
function [T1, T2, T3] = fcn(q1, qd1, qdd1, q2, qd2, qdd2, q3, qd3, qdd3)

l1 = 0.0285; l2 = 0.0758; l3 = 0.1298;
%q1 = 2; q2 = 0; q3 = pi/8;
%qd1 = 0.1; qd2 = 0.1; qd3 = 0.1;
%qdd1 = 0.1; qdd1 = 9; qdd1 = 0.01;
lc1 = l1/2; lc2 = l2/2; lc3 = l3/2;

Ixx1 = 0.000; Ixx2 = 0.000; Ixx3 = 0.000;
Iyy1 = 0.000; Iyy2 = 0.000; Iyy3 = 0.000;
Izz1 = 0.000; Izz2 = 0.000; Izz3 = 0.0000;

gx = 0;
gy = 0;
gz = 9.81;
m1 = 2; m2 = 2; m3 = 2;

Fx = 0;
Fy = 0;
Fz = 0;
b1 = 0.1; b2 = 0.1; b3 = 0.1; 


T1 = (Ixx2*qdd1)/2 - Fz*l1 + (Ixx3 * qdd1)/2 + Iyy1*qdd1 + (Iyy2*qdd1)/2 + (Iyy3*qdd1)/2 + b1*qd1 + l1^2*m2*qdd1 + l1^2*m3*qdd1 + (l2^2*m3*qdd1)/2 + lc1^2*m1*qdd1 + (lc2^2*m2*qdd1)/2 + (lc3^2*m3*qdd1)/2 - (Ixx2*qdd1*cos(2*q2))/2 + (Iyy2*qdd1*cos(2*q2))/2 - (Ixx3*qdd1*cos(2*q2 + 2*q3))/2 + (Iyy3*qdd1*cos(2*q2 + 2*q3))/2 - Fz*l3*cos(q2 + q3) - Fz*l2*cos(q2) + (gy*lc3*m3*cos(q2 - q1 + q3))/2 + (gx*lc3*m3*sin(q2 - q1 + q3))/2 + (l2^2*m3*qdd1*cos(2*q2))/2 + (lc2^2*m2*qdd1*cos(2*q2))/2 + (gy*l2*m3*cos(q1 + q2))/2 + (gy*lc2*m2*cos(q1 + q2))/2 - (gx*l2*m3*sin(q1 + q2))/2 - (gx*lc2*m2*sin(q1 + q2))/2 + (lc3^2*m3*qdd1*cos(2*q2 + 2*q3))/2 + gy*l1*m2*cos(q1) + gy*l1*m3*cos(q1) + gy*lc1*m1*cos(q1) - gx*l1*m2*sin(q1) - gx*l1*m3*sin(q1) - gx*lc1*m1*sin(q1) + (gy*l2*m3*cos(q1 - q2))/2 + (gy*lc2*m2*cos(q1 - q2))/2 - (gx*l2*m3*sin(q1 - q2))/2 - (gx*lc2*m2*sin(q1 - q2))/2 + (gy*lc3*m3*cos(q1 + q2 + q3))/2 - (gx*lc3*m3*sin(q1 + q2 + q3))/2 + Ixx2*qd1*qd2*sin(2*q2) - Iyy2*qd1*qd2*sin(2*q2) + Ixx3*qd1*qd2*sin(2*q2 + 2*q3) + Ixx3*qd1*qd3*sin(2*q2 + 2*q3) - Iyy3*qd1*qd2*sin(2*q2 + 2*q3) - Iyy3*qd1*qd3*sin(2*q2 + 2*q3) + l2*lc3*m3*qdd1*cos(2*q2 + q3) + 2*l1*lc3*m3*qdd1*cos(q2 + q3) - l2^2*m3*qd1*qd2*sin(2*q2) - lc2^2*m2*qd1*qd2*sin(2*q2) + 2*l1*l2*m3*qdd1*cos(q2) + 2*l1*lc2*m2*qdd1*cos(q2) + l2*lc3*m3*qdd1*cos(q3) - lc3^2*m3*qd1*qd2*sin(2*q2 + 2*q3) - lc3^2*m3*qd1*qd3*sin(2*q2 + 2*q3) - 2*l1*lc3*m3*qd1*qd2*sin(q2 + q3) - 2*l1*lc3*m3*qd1*qd3*sin(q2 + q3) - 2*l1*l2*m3*qd1*qd2*sin(q2) - 2*l1*lc2*m2*qd1*qd2*sin(q2) - l2*lc3*m3*qd1*qd3*sin(q3) - 2*l2*lc3*m3*qd1*qd2*sin(2*q2 + q3) - l2*lc3*m3*qd1*qd3*sin(2*q2 + q3);
T2 = Fy*l3 + Izz2*qdd2 + Izz3*qdd2 + Izz3*qdd3 + b2*qd2 + l2^2*m3*qdd2 + lc2^2*m2*qdd2 + lc3^2*m3*qdd2 + lc3^2*m3*qdd3 - (Ixx2*qd1^2*sin(2*q2))/2 + (Iyy2*qd1^2*sin(2*q2))/2 + Fy*l2*cos(q3) - (Ixx3*qd1^2*sin(2*q2 + 2*q3))/2 + (Iyy3*qd1^2*sin(2*q2 + 2*q3))/2 + Fx*l2*sin(q3) - (gy*lc3*m3*cos(q2 - q1 + q3))/2 - (gx*lc3*m3*sin(q2 - q1 + q3))/2 + (gy*l2*m3*cos(q1 + q2))/2 + (gy*lc2*m2*cos(q1 + q2))/2 + gz*lc3*m3*cos(q2 + q3) - (gx*l2*m3*sin(q1 + q2))/2 - (gx*lc2*m2*sin(q1 + q2))/2 + gz*l2*m3*cos(q2) + gz*lc2*m2*cos(q2) - (gy*l2*m3*cos(q1 - q2))/2 - (gy*lc2*m2*cos(q1 - q2))/2 + (l2^2*m3*qd1^2*sin(2*q2))/2 + (lc2^2*m2*qd1^2*sin(2*q2))/2 + (gx*l2*m3*sin(q1 - q2))/2 + (gx*lc2*m2*sin(q1 - q2))/2 + (gy*lc3*m3*cos(q1 + q2 + q3))/2 - (gx*lc3*m3*sin(q1 + q2 + q3))/2 + (lc3^2*m3*qd1^2*sin(2*q2 + 2*q3))/2 + l1*lc3*m3*qd1^2*sin(q2 + q3) + l1*l2*m3*qd1^2*sin(q2) + l1*lc2*m2*qd1^2*sin(q2) - l2*lc3*m3*qd3^2*sin(q3) + l2*lc3*m3*qd1^2*sin(2*q2 + q3) + 2*l2*lc3*m3*qdd2*cos(q3) + l2*lc3*m3*qdd3*cos(q3) - 2*l2*lc3*m3*qd2*qd3*sin(q3);
T3 = Fy*l3 + Izz3*qdd2 + Izz3*qdd3 + b3*qd3 + lc3^2*m3*qdd2 + lc3^2*m3*qdd3 - (Ixx3*qd1^2*sin(2*q2 + 2*q3))/2 + (Iyy3*qd1^2*sin(2*q2 + 2*q3))/2 - (gy*lc3*m3*cos(q2 - q1 + q3))/2 - (gx*lc3*m3*sin(q2 - q1 + q3))/2 + gz*lc3*m3*cos(q2 + q3) + (gy*lc3*m3*cos(q1 + q2 + q3))/2 - (gx*lc3*m3*sin(q1 + q2 + q3))/2 + (lc3^2*m3*qd1^2*sin(2*q2 + 2*q3))/2 + l1*lc3*m3*qd1^2*sin(q2 + q3) + (l2*lc3*m3*qd1^2*sin(q3))/2 + l2*lc3*m3*qd2^2*sin(q3) + (l2*lc3*m3*qd1^2*sin(2*q2 + q3))/2 + l2*lc3*m3*qdd2*cos(q3);

== matlab function hex_simplify_mono/N(theta,dtheta)/MATLAB Function1 ==
  data: q1 input; N1 output; q2 input; N2 output; N3 output; q3 input; qd1 input; qd2 input; qd3 input
function [N1, N2, N3] = fcn(q1,q2,q3,qd1,qd2,qd3)


l1 = 0.0285; l2 = 0.0758; l3 = 0.1298;
%q1 = 2; q2 = 0; q3 = pi/8;
%qd1 = 0.1; qd2 = 0.1; qd3 = 0.1;
%qdd1 = 0.1; qdd1 = 9; qdd1 = 0.01;
lc1 = l1/2; lc2 = l2/2; lc3 = l3/2;

Ixx1 = 0.000; Ixx2 = 0.000; Ixx3 = 0.000;
Iyy1 = 0.000; Iyy2 = 0.000; Iyy3 = 0.000;
Izz1 = 0.000; Izz2 = 0.000; Izz3 = 0.0000;

gx = 0;
gy = 0;
gz = 9.81;
m1 = 2; m2 = 2; m3 = 2;

Fx = 0;
Fy = 0;
Fz = 0;
b1 = 0.1; b2 = 0.1; b3 = 0.1; 

N1 = - Fz*l1  + b1*qd1 - Fz*l3*cos(q2 + q3) - Fz*l2*cos(q2) + (gy*lc3*m3*cos(q2 - q1 + q3))/2 + (gx*lc3*m3*sin(q2 - q1 + q3))/2 + (gy*l2*m3*cos(q1 + q2))/2 + (gy*lc2*m2*cos(q1 + q2))/2 - (gx*l2*m3*sin(q1 + q2))/2 - (gx*lc2*m2*sin(q1 + q2))/2 + gy*l1*m2*cos(q1) + gy*l1*m3*cos(q1) + gy*lc1*m1*cos(q1) - gx*l1*m2*sin(q1) - gx*l1*m3*sin(q1) - gx*lc1*m1*sin(q1) + (gy*l2*m3*cos(q1 - q2))/2 + (gy*lc2*m2*cos(q1 - q2))/2 - (gx*l2*m3*sin(q1 - q2))/2 - (gx*lc2*m2*sin(q1 - q2))/2 + (gy*lc3*m3*cos(q1 + q2 + q3))/2 - (gx*lc3*m3*sin(q1 + q2 + q3))/2 + Ixx2*qd1*qd2*sin(2*q2) - Iyy2*qd1*qd2*sin(2*q2) + Ixx3*qd1*qd2*sin(2*q2 + 2*q3) + Ixx3*qd1*qd3*sin(2*q2 + 2*q3) - Iyy3*qd1*qd2*sin(2*q2 + 2*q3) - Iyy3*qd1*qd3*sin(2*q2 + 2*q3)  - l2^2*m3*qd1*qd2*sin(2*q2) - lc2^2*m2*qd1*qd2*sin(2*q2)   - lc3^2*m3*qd1*qd2*sin(2*q2 + 2*q3) - lc3^2*m3*qd1*qd3*sin(2*q2 + 2*q3) - 2*l1*lc3*m3*qd1*qd2*sin(q2 + q3) - 2*l1*lc3*m3*qd1*qd3*sin(q2 + q3) - 2*l1*l2*m3*qd1*qd2*sin(q2) - 2*l1*lc2*m2*qd1*qd2*sin(q2) - l2*lc3*m3*qd1*qd3*sin(q3) - 2*l2*lc3*m3*qd1*qd2*sin(2*q2 + q3) - l2*lc3*m3*qd1*qd3*sin(2*q2 + q3);
N2 = Fy*l3 + b2*qd2 - (Ixx2*qd1^2*sin(2*q2))/2 + (Iyy2*qd1^2*sin(2*q2))/2 + Fy*l2*cos(q3) - (Ixx3*qd1^2*sin(2*q2 + 2*q3))/2 + (Iyy3*qd1^2*sin(2*q2 + 2*q3))/2 + Fx*l2*sin(q3) - (gy*lc3*m3*cos(q2 - q1 + q3))/2 - (gx*lc3*m3*sin(q2 - q1 + q3))/2 + (gy*l2*m3*cos(q1 + q2))/2 + (gy*lc2*m2*cos(q1 + q2))/2 + gz*lc3*m3*cos(q2 + q3) - (gx*l2*m3*sin(q1 + q2))/2 - (gx*lc2*m2*sin(q1 + q2))/2 + gz*l2*m3*cos(q2) + gz*lc2*m2*cos(q2) - (gy*l2*m3*cos(q1 - q2))/2 - (gy*lc2*m2*cos(q1 - q2))/2 + (l2^2*m3*qd1^2*sin(2*q2))/2 + (lc2^2*m2*qd1^2*sin(2*q2))/2 + (gx*l2*m3*sin(q1 - q2))/2 + (gx*lc2*m2*sin(q1 - q2))/2 + (gy*lc3*m3*cos(q1 + q2 + q3))/2 - (gx*lc3*m3*sin(q1 + q2 + q3))/2 + (lc3^2*m3*qd1^2*sin(2*q2 + 2*q3))/2 + l1*lc3*m3*qd1^2*sin(q2 + q3) + l1*l2*m3*qd1^2*sin(q2) + l1*lc2*m2*qd1^2*sin(q2) - l2*lc3*m3*qd3^2*sin(q3) + l2*lc3*m3*qd1^2*sin(2*q2 + q3) - 2*l2*lc3*m3*qd2*qd3*sin(q3);
N3 = Fy*l3 + b3*qd3 - (Ixx3*qd1^2*sin(2*q2 + 2*q3))/2 + (Iyy3*qd1^2*sin(2*q2 + 2*q3))/2 - (gy*lc3*m3*cos(q2 - q1 + q3))/2 - (gx*lc3*m3*sin(q2 - q1 + q3))/2 + gz*lc3*m3*cos(q2 + q3) + (gy*lc3*m3*cos(q1 + q2 + q3))/2 - (gx*lc3*m3*sin(q1 + q2 + q3))/2 + (lc3^2*m3*qd1^2*sin(2*q2 + 2*q3))/2 + l1*lc3*m3*qd1^2*sin(q2 + q3) + (l2*lc3*m3*qd1^2*sin(q3))/2 + l2*lc3*m3*qd2^2*sin(q3) + (l2*lc3*m3*qd1^2*sin(2*q2 + q3))/2 ;
